simulink model "pm4_motor_func"  (R2017a)
settings: Solver=VariableStepAuto  StartTime=0.0  StopTime=10.0  RelTol=1e-3
libraries: simulink x1
settings Model: Creator=robotica  LastModifiedBy=robotica

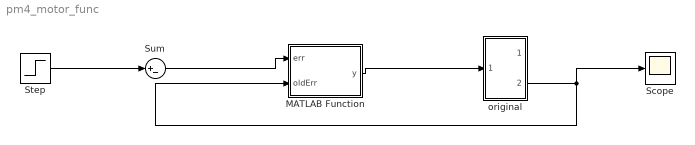
== system pm4_motor_func ==
  MATLAB Function : MATLAB Function  TreatAsAtomicUnit=on
  Scope : Scope
  Step : Step  SampleTime=1
  Sum : Sum  Inputs=|+-
  original : Subsystem
  wires:
  MATLAB Function/1(y) -> original/1(signal)
  Sum/1 -> MATLAB Function/1(err)
  original/2(clean) -> MATLAB Function/2(oldErr), Scope/1
  Step/1 -> Sum/1

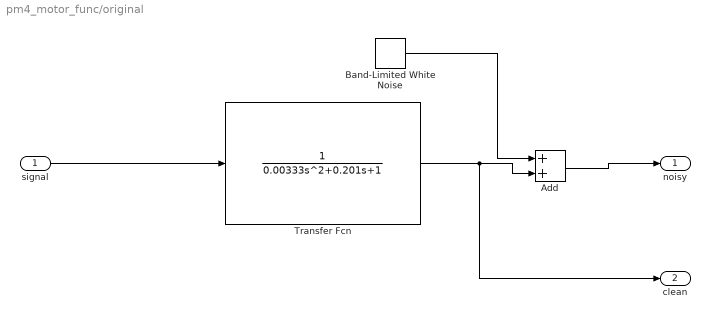
== system pm4_motor_func/original ==
  signal : Inport
  Add : Sum
  Band-Limited White Noise : simulink/Sources/Band-Limited White Noise  Cov=[0.0000001]  Ts=0.001  seed=[23341]
  Transfer Fcn : TransferFcn  Denominator=[0.00333 0.201 1]
  noisy : Outport
  clean : Outport  Port=2
  wires:
  Transfer Fcn/1 -> clean/1, Add/2
  Band-Limited White Noise/1 -> Add/1
  Add/1 -> noisy/1
  signal/1 -> Transfer Fcn/1

== matlab function pm4_motor_func/MATLAB Function ==
  data: err input; y output; oldErr input
function y = fcn(err, oldErr)
kp = 25;
ki = 20;
kd = 0.375;

gain1 = err * kp;
gain2 = err * ki;
gain2
gain3 = kd * err;

y = gain1 + gain2 + gain3;
